simulink model "Projekt2_ACC"  (R2023a)
settings: Solver=FixedStepAuto  StartTime=0.0  StopTime=60  RelTol=1e-3
undefined symbols (not defined in the file): LF
libraries: instrumentseriallib x2, slpidlib x1
settings Model: Creator=karim  LastModifiedBy=karim

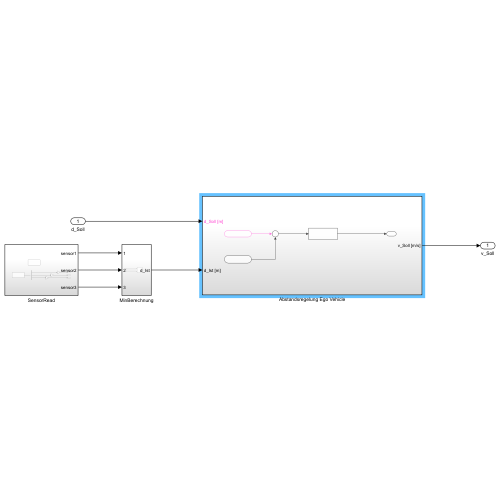
[thumbnail: Simulink's stored preview of the top-level diagram]
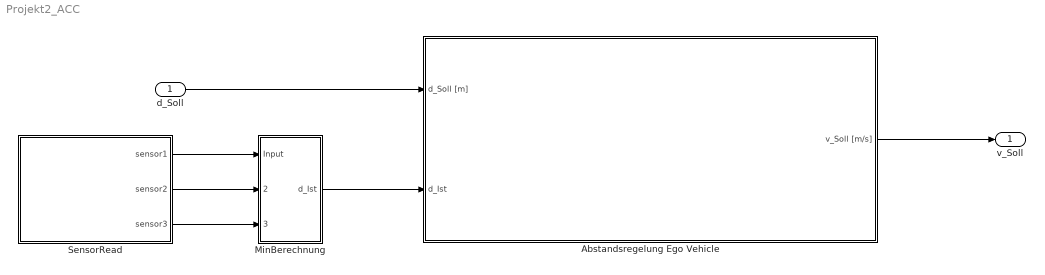
== system Projekt2_ACC ==
  d_Soll : Inport
  Abstandsregelung Ego Vehicle : Subsystem
  MinBerechnung : Subsystem
  SensorRead : Subsystem
  v_Soll : Outport
  wires:
  SensorRead/3(sensor3) -> MinBerechnung/3(Input2)
  SensorRead/2(sensor2) -> MinBerechnung/2(Input1)
  SensorRead/1(sensor1) -> MinBerechnung/1(Input)
  d_Soll/1 -> Abstandsregelung Ego Vehicle/1(d_Soll [m])
  Abstandsregelung Ego Vehicle/1(v_Soll [m/s]) -> v_Soll/1
  MinBerechnung/1(d_Ist) -> Abstandsregelung Ego Vehicle/2(d_Ist)

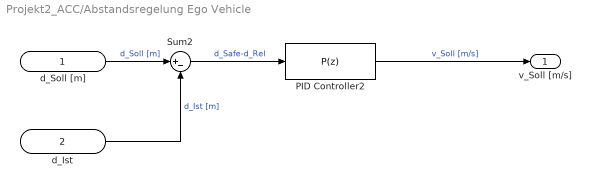
== system Projekt2_ACC/Abstandsregelung Ego Vehicle ==
  d_Soll [m] : Inport
  d_Ist : Inport  Port=2
  PID Controller2 : slpidlib/PID Controller  Controller=P  Form=Parallel  TimeDomain=Discrete-time  UseExternalTs=off  SampleTime=-1  IntegratorMethod=Forward Euler  FilterMethod=Forward Euler  ControllerParametersSource=internal  P=30  I=3  UseKiTs=off  D=-20  N=1  UseFilter=off  TunerSelectOption=Transfer Function Based (PID Tuner App)  InitialConditionSource=internal  InitialConditionForIntegrator=0  InitialConditionForFilter=0  DifferentiatorICPrevScaledInput=0  ExternalReset=none  TrackingMode=off  Kt=1  LimitOutput=on  SatLimitsSource=internal  UpperSaturationLimit=60  LowerSaturationLimit=-60  LinearizeAsGain=on  AntiWindupMode=clamping  Kb=1  LimitIntegrator=off  UpperIntegratorSaturationLimit=inf  LowerIntegratorSaturationLimit=-inf  POutMin=[]  POutMax=[]  IOutMin=[]  IOutMax=[]  DOutMin=[]  DOutMax=[]  NOutMin=[]  NOutMax=[]  SumOutMin=[]  SumOutMax=[]  SaturationOutMin=[]  SaturationOutMax=[]  PParamMin=[]  PParamMax=[]  IParamMin=[]  IParamMax=[]  DParamMin=[]  DParamMax=[]  NParamMin=[]  NParamMax=[]  KbParamMin=[]  KbParamMax=[]  KtParamMin=[]  KtParamMax=[]  KbOutMin=[]  KbOutMax=[]  KtOutMin=[]  KtOutMax=[]  IntegratorOutMin=[]  IntegratorOutMax=[]  FilterOutMin=[]  FilterOutMax=[]  SumI1OutMin=[]  SumI1OutMax=[]  SumI2OutMin=[]  SumI2OutMax=[]  SumI3OutMin=[]  SumI3OutMax=[]  SumI4OutMin=[]  SumI4OutMax=[]  SumDOutMin=[]  SumDOutMax=[]  DifferentiatorOutMin=[]  DifferentiatorOutMax=[]  FilterDiffOutCoefMin=[]  FilterDiffOutCoefMax=[]  ReciprocalOutMin=[]  ReciprocalOutMax=[]  SumDenOutMin=[]  SumDenOutMax=[]  SumNumOutMin=[]  SumNumOutMax=[]  DivideOutMin=[]  DivideOutMax=[]  UdiffTsProdOutMin=[]  UdiffTsProdOutMax=[]  NTsProdOutMin=[]  NTsProdOutMax=[]  UintegralTsProdOutMin=[]  UintegralTsProdOutMax=[]  UngainTsProdOutMin=[]  UngainTsProdOutMax=[]  ClampingZeroOutDataTypeStr=Inherit: Inherit via back propagation  ClampingZeroOutMin=[]  ClampingZeroOutMax=[]  FilterDenConstantOutDataTypeStr=Inherit: Inherit via back propagation  FilterDenConstantOutMin=[]  FilterDenConstantOutMax=[]  PCopyOutDataTypeStr=Inherit: Inherit via back propagation  PCopyOutMin=[]  PCopyOutMax=[]  NCopyOutDataTypeStr=Inherit: Inherit via back propagation  NCopyOutMin=[]  NCopyOutMax=[]  IntegratorContinuousStateAttributes=''  IntegratorStateMustResolveToSignalObject=off  IntegratorRTWStateStorageClass=Auto  FilterContinuousStateAttributes=''  FilterStateMustResolveToSignalObject=off  FilterRTWStateStorageClass=Auto  ParallelPVariant=InternalParameters  IdealPVariant=Disabled  IVariant=Disabled  DVariant=Disabled  IntegratorVariant=Disabled  SatVariant=Enabled  AWVariant=Disabled  PCopyVariant=Disabled  TRVariant=Disabled  FdbkBlocksVariant=Forward  IdealPFdbkVariant=Disabled  SatFdbkVariant=Disabled  DerivativeFilterVariant=Disabled  NVariant=Disabled  NCopyVariant=Disabled_SignalSpec  FilterICVariant=Disabled  IntegratorICVariant=Disabled  ExternalResetVariant=Disabled  TRSumVariant=Passthrough  SumFdbkVariant=Disabled  SumVariant=Passthrough_P  TsampFilterVariant=InternalTs  TsampNgainVariant=Passthrough  TsampIntegralVariant=Disabled_SignalSpec  ExternalSaturationOutDataTypeStr=Inherit: Same as second input
  Sum2 : Sum  Inputs=|+-
  v_Soll [m/s] : Outport
  wires:
  d_Soll [m]/1 -> Sum2/1  "d_Soll [m]"
  Sum2/1 -> PID Controller2/1  "d_Safe-d_Rel"
  d_Ist/1 -> Sum2/2  "d_Ist [m]"
  PID Controller2/1 -> v_Soll [m/s]/1  "v_Soll [m/s]"

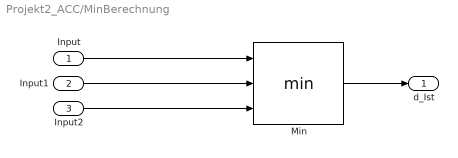
== system Projekt2_ACC/MinBerechnung ==
  Input : Inport
  Input1 : Inport  Port=2
  Input2 : Inport  Port=3
  Min : MinMax  Inputs=3
  d_Ist : Outport
  wires:
  Input/1 -> Min/1
  Input1/1 -> Min/2
  Input2/1 -> Min/3
  Min/1 -> d_Ist/1

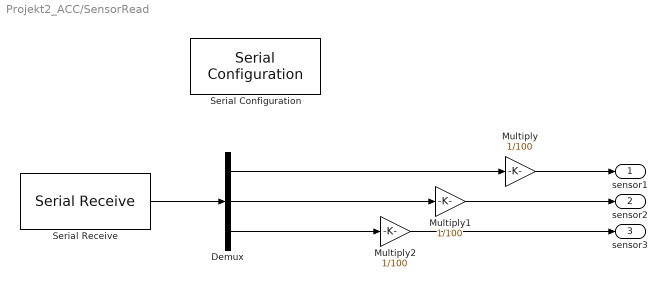
== system Projekt2_ACC/SensorRead ==
  Demux : Demux  Outputs=3
  Multiply : Gain  Gain=1/100
  Multiply1 : Gain  Gain=1/100
  Multiply2 : Gain  Gain=1/100
  Serial Configuration : instrumentseriallib/Serial Configuration  Priority=-200000  PortSel=COM7  Port=COM7  ComPort=COM7  BaudRate=115200  DataBits=8  Parity=none  StopBits=1  ByteOrder=little-endian  FlowControl=none  Timeout=10  SimulateUsing=Interpreted execution  BlockInModel=on  aMode=1
  Serial Receive : instrumentseriallib/Serial Receive  Priority=1  PortSel=COM7  Port=COM7  ComPort=COM7  DataType=single  SaveDataType=uint8  ToggleHeader=on  Header=[65]  ToggleTerminator=on  Terminator=LF ('\n')  CustomTerminator=[]  InputFormat=Column major  ToggleDataSize=on  DataSize=[1 3]  EnableBlockingMode=on  ActionDataUnavailable=Output last received value  ActionWhenDataUnavailable=Output last received value  CustomValue=0  SampleTime=0.05  SimulateUsing=Interpreted execution  BlockInModel=on  aMode=1
  sensor1 : Outport
  sensor2 : Outport  Port=2
  sensor3 : Outport  Port=3
  wires:
  Demux/3 -> Multiply2/1
  Serial Receive/1 -> Demux/1
  Demux/2 -> Multiply1/1
  Demux/1 -> Multiply/1
  Multiply2/1 -> sensor3/1
  Multiply1/1 -> sensor2/1
  Multiply/1 -> sensor1/1
